simulink model "aux_test"  (R2022b)
settings: Solver=VariableStepAuto  StartTime=0.0  StopTime=10.0  RelTol=1e-3
settings Model: Creator=dding  LastModifiedBy=dding

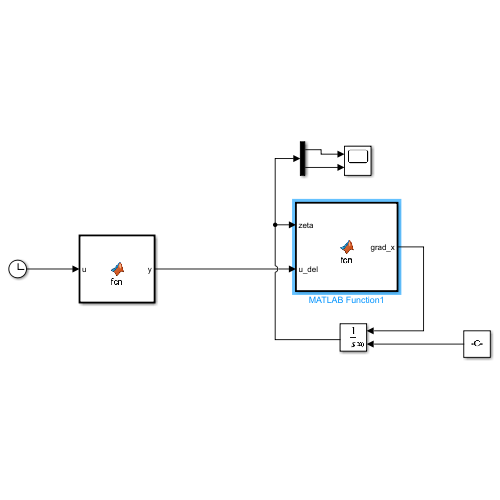
[thumbnail: Simulink's stored preview of the top-level diagram]
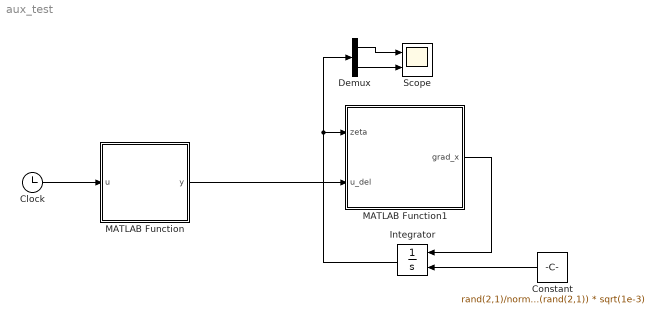
== system aux_test ==
  Clock : Clock
  Constant : Constant  Value=rand(2,1)/norm(rand(2,1)) * sqrt(1e-3)
  Demux : Demux  Outputs=2
  Integrator : Integrator  InitialConditionSource=external
  MATLAB Function : MATLAB Function  TreatAsAtomicUnit=on
  MATLAB Function1 : MATLAB Function  TreatAsAtomicUnit=on
  Scope : Scope  NumInputPorts=2
  wires:
  MATLAB Function/1(y) -> MATLAB Function1/2(u_del)
  MATLAB Function1/1(grad_x) -> Integrator/1
  Integrator/1 -> Demux/1, MATLAB Function1/1(zeta)
  Clock/1 -> MATLAB Function/1(u)
  Constant/1 -> Integrator/2
  Demux/1 -> Scope/1
  Demux/2 -> Scope/2

== matlab function aux_test/MATLAB Function ==
  data: u input; y output
function y = fcn(u)

y = [50 * sin(u); 50 * cos(u)];

== matlab function aux_test/MATLAB Function1 ==
  data: zeta input; grad_x output; u_del input
function grad_x = fcn(zeta, u_del)

Kzeta = 1e5;
mu = 1e-3;
e2 = [0.1; 1];
if norm(zeta) >= sqrt(mu)
    grad_x = -Kzeta * zeta - ( abs(e2'*u_del)+0.5*u_del'*u_del )/ norm(zeta)^2 * zeta + u_del;
else
    grad_x = zeros(size(zeta));
end
